simulink model "LQR_Implementation"  (R2018b)
settings: Solver=VariableStepAuto  StartTime=0.0  StopTime=10  RelTol=1e-10
values from neighbouring files (symbols this model uses):
  Ad = [0.9970    0.0020    0.0021   -0.0019 ... (first row only)    [LQRDesign.m]    (also in LQR_Design.m; MPCDesign.m; MPC_Design.m; modelEstimation.m = [Theta1(1:4,1).')
  Bd = [-0.0000    0.0000 ... (first row only)    [LQRDesign.m]    (also in LQR_Design.m; MPCDesign.m; MPC_Design.m; modelEstimation.m = [Theta1(5:6,1).')
  Cd = [1.0000         0         0         0 ... (first row only)    [LQRDesign.m]    (also in LQR_Design.m; MPCDesign.m; MPC_Design.m; modelEstimation.m = [1 0 0 0)
  Dd = [0   0 ... (first row only)    [LQRDesign.m]    (also in LQR_Design.m; MPCDesign.m; MPC_Design.m; modelEstimation.m = [0 0)
  T = 0.002    [LQRDesign.m]    (also in LQR_Design.m; MPCDesign.m; MPC_Design.m; dataProcessing.m)
undefined symbols (not defined in the file or in its folder): K1, K2, K3, K4
libraries: simulink x10
settings Model: Creator=oxyoung  LastModifiedBy=Administrator

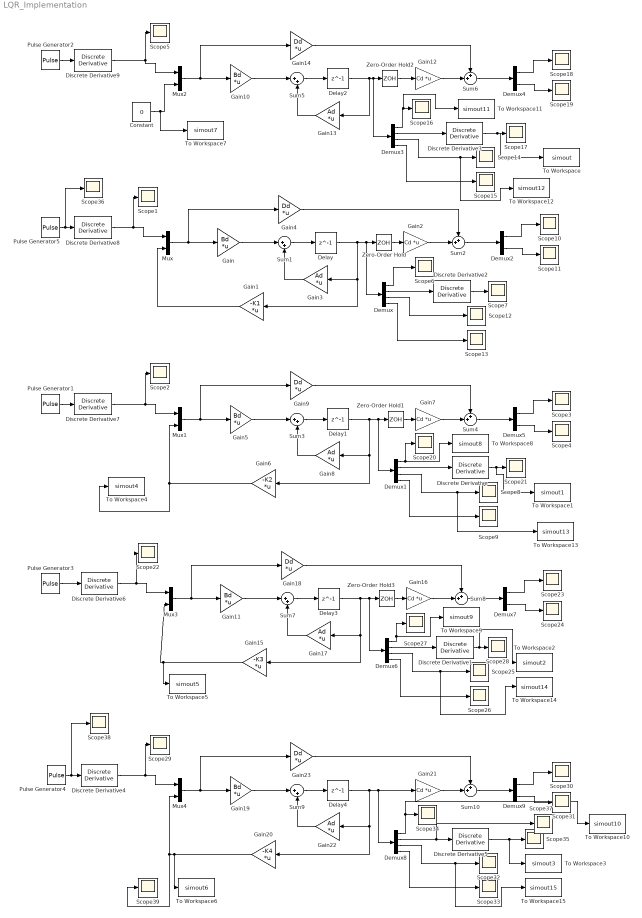
== system LQR_Implementation ==
  Constant : Constant  Value=0
  Delay{,1..4} (5 alike) : Delay  DelayLength=1  SampleTime=T
  Demux{,1,3,6,8} (5 alike) : Demux
  Demux{2,4..5,7,9} (5 alike) : Demux  Outputs=2
  Discrete Derivative{,1..9} (10 alike) : simulink/Quick Insert/Discrete/Discrete Derivative  gainval=1.0  ICPrevScaledInput=0.0  OutMin=[]  OutMax=[]  OutDataType=fixdt(1, 16)  OutScaling=2^-10  DoSatur=off
      settings: SourceProductName=Simulink  SourceProductBaseCode=SL
  Gain{,5,10..11,19} (5 alike) : Gain  Gain=Bd  Multiplication=Matrix(K*u)
  Gain1 : Gain  Gain=-K1  Multiplication=Matrix(K*u)
  Gain{2,7,12,16,21} (5 alike) : Gain  Gain=Cd  Multiplication=Matrix(K*u)
  Gain{3,8,13,17,22} (5 alike) : Gain  Gain=Ad  Multiplication=Matrix(K*u)
  Gain{4,9,14,18,23} (5 alike) : Gain  Gain=Dd  Multiplication=Matrix(K*u)
  Gain15 : Gain  Gain=-K3  Multiplication=Matrix(K*u)
  Gain20 : Gain  Gain=-K4  Multiplication=Matrix(K*u)
  Gain6 : Gain  Gain=-K2  Multiplication=Matrix(K*u)
  Mux{,1..4} (5 alike) : Mux  Inputs=2
  Pulse Generator{1..5} (5 alike) : DiscretePulseGenerator  PulseType=Time based  Amplitude=0.01  Period=1/0.3  PulseWidth=20
  Scope{1..39} (39 alike) : Scope
  Sum{1,3,5,7,9} (5 alike) : Sum  Inputs=|++
  Sum{2,4,6,8,10} (5 alike) : Sum  Inputs=++|
  To Workspace : ToWorkspace  VariableName=simout  SaveFormat=Structure With Time  SampleTime=-1
  To Workspace1 : ToWorkspace  VariableName=simout1  SaveFormat=Structure With Time  SampleTime=-1
  To Workspace10 : ToWorkspace  VariableName=simout10  SaveFormat=Structure With Time  SampleTime=-1
  To Workspace11 : ToWorkspace  VariableName=simout11  SaveFormat=Structure With Time  SampleTime=-1
  To Workspace12 : ToWorkspace  VariableName=simout12  SaveFormat=Structure With Time  SampleTime=-1
  To Workspace13 : ToWorkspace  VariableName=simout13  SaveFormat=Structure With Time  SampleTime=-1
  To Workspace14 : ToWorkspace  VariableName=simout14  SaveFormat=Structure With Time  SampleTime=-1
  To Workspace15 : ToWorkspace  VariableName=simout15  SaveFormat=Structure With Time  SampleTime=-1
  To Workspace2 : ToWorkspace  VariableName=simout2  SaveFormat=Structure With Time  SampleTime=-1
  To Workspace3 : ToWorkspace  VariableName=simout3  SaveFormat=Structure With Time  SampleTime=-1
  To Workspace4 : ToWorkspace  VariableName=simout4  SaveFormat=Structure With Time  SampleTime=-1
  To Workspace5 : ToWorkspace  VariableName=simout5  SaveFormat=Structure With Time  SampleTime=-1
  To Workspace6 : ToWorkspace  VariableName=simout6  SaveFormat=Structure With Time  SampleTime=-1
  To Workspace7 : ToWorkspace  VariableName=simout7  SaveFormat=Structure With Time  SampleTime=-1
  To Workspace8 : ToWorkspace  VariableName=simout8  SaveFormat=Structure With Time  SampleTime=-1
  To Workspace9 : ToWorkspace  VariableName=simout9  SaveFormat=Structure With Time  SampleTime=-1
  Zero-Order Hold{,1..3} (4 alike) : ZeroOrderHold  SampleTime=0.002
  wires:
  Mux/1 -> Gain/1, Gain4/1
  Sum1/1 -> Delay/1
  Gain1/1 -> Mux/2
  Gain3/1 -> Sum1/2
  Delay/1 -> Demux/1, Zero-Order Hold/1, Gain1/1, Gain3/1
  Gain/1 -> Sum1/1
  Zero-Order Hold/1 -> Gain2/1
  Gain4/1 -> Sum2/1
  Gain2/1 -> Sum2/2
  Discrete Derivative8/1 -> Scope1/1, Mux/1
  Sum5/1 -> Delay2/1
  Mux2/1 -> Gain10/1, Gain14/1
  Gain12/1 -> Sum6/2
  Gain14/1 -> Sum6/1
  Gain13/1 -> Sum5/2
  Zero-Order Hold2/1 -> Gain12/1
  Discrete Derivative9/1 -> Mux2/1, Scope5/1
  Gain10/1 -> Sum5/1
  Constant/1 -> To Workspace7/1, Mux2/2
  Demux/1 -> Scope6/1
  Demux/2 -> Discrete Derivative2/1
  Discrete Derivative2/1 -> Scope7/1
  Sum2/1 -> Demux2/1
  Demux2/1 -> Scope10/1
  Demux2/2 -> Scope11/1
  Demux/3 -> Scope12/1
  Demux/4 -> Scope13/1
  Discrete Derivative3/1 -> To Workspace/1, Scope17/1
  Demux3/3 -> To Workspace12/1, Scope14/1
  Demux3/4 -> Scope15/1
  Demux3/1 -> To Workspace11/1, Scope16/1
  Delay2/1 -> Demux3/1, Zero-Order Hold2/1, Gain13/1
  Demux3/2 -> Discrete Derivative3/1
  Demux4/1 -> Scope18/1
  Sum6/1 -> Demux4/1
  Demux4/2 -> Scope19/1
  Demux5/1 -> Scope3/1
  Sum4/1 -> Demux5/1
  Demux5/2 -> Scope4/1
  Demux1/3 -> To Workspace13/1, Scope8/1
  Discrete Derivative/1 -> To Workspace1/1, Scope21/1
  Gain5/1 -> Sum3/1
  Gain7/1 -> Sum4/2
  Zero-Order Hold1/1 -> Gain7/1
  Gain6/1 -> To Workspace4/1, Mux1/2
  Delay1/1 -> Demux1/1, Zero-Order Hold1/1, Gain6/1, Gain8/1
  Mux1/1 -> Gain5/1, Gain9/1
  Discrete Derivative7/1 -> Scope2/1, Mux1/1
  Demux1/4 -> Scope9/1
  Demux1/1 -> Scope20/1, To Workspace8/1
  Sum3/1 -> Delay1/1
  Demux1/2 -> Discrete Derivative/1
  Gain8/1 -> Sum3/2
  Gain9/1 -> Sum4/1
  Demux7/1 -> Scope23/1
  Sum8/1 -> Demux7/1
  Demux7/2 -> Scope24/1
  Demux6/3 -> To Workspace14/1, Scope25/1
  Discrete Derivative1/1 -> To Workspace2/1, Scope28/1
  Gain11/1 -> Sum7/1
  Gain16/1 -> Sum8/2
  Pulse Generator3/1 -> Discrete Derivative6/1
  Zero-Order Hold3/1 -> Gain16/1
  Gain15/1 -> To Workspace5/1, Mux3/2
  Delay3/1 -> Demux6/1, Zero-Order Hold3/1, Gain15/1, Gain17/1
  Mux3/1 -> Gain11/1, Gain18/1
  Discrete Derivative6/1 -> Scope22/1, Mux3/1
  Demux6/4 -> Scope26/1
  Demux6/1 -> To Workspace9/1, Scope27/1
  Sum7/1 -> Delay3/1
  Demux6/2 -> Discrete Derivative1/1
  Gain17/1 -> Sum7/2
  Gain18/1 -> Sum8/1
  Demux9/1 -> Scope30/1
  Sum10/1 -> Demux9/1
  Demux9/2 -> Scope31/1
  Demux8/3 -> To Workspace15/1, Scope32/1
  Discrete Derivative5/1 -> To Workspace3/1, Scope35/1
  Gain19/1 -> Sum9/1
  Gain21/1 -> Sum10/2
  Pulse Generator4/1 -> Scope38/1, Discrete Derivative4/1
  Delay4/1 -> Gain21/1, Demux8/1, Gain20/1, Gain22/1
  Gain20/1 -> To Workspace6/1, Mux4/2, Scope39/1
  Mux4/1 -> Gain19/1, Gain23/1
  Discrete Derivative4/1 -> Scope29/1, Mux4/1
  Demux8/4 -> Scope33/1
  Demux8/1 -> To Workspace10/1, Scope34/1
  Sum9/1 -> Delay4/1
  Demux8/2 -> Scope37/1, Discrete Derivative5/1
  Gain22/1 -> Sum9/2
  Gain23/1 -> Sum10/1
  Pulse Generator1/1 -> Discrete Derivative7/1
  Pulse Generator5/1 -> Scope36/1, Discrete Derivative8/1
  Pulse Generator2/1 -> Discrete Derivative9/1
